simulink model "Function11"  (R2016b)
settings: Solver=VariableStepAuto  StartTime=0.0  StopTime=10.0  RelTol=1e-3
libraries: simulink x2
settings Model: Creator=viett  LastModifiedBy=viett

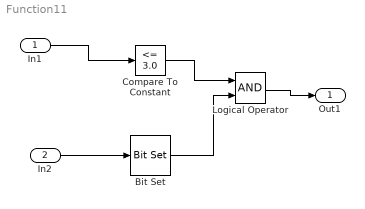
== system Function11 ==
  In1 : Inport
  In2 : Inport  Port=2
  Bit Set : simulink/Logic and Bit Operations/Bit Set  iBit=0
  Compare To Constant : simulink/Logic and Bit Operations/Compare To Constant  relop=<=  const=3.0  OutDataTypeStr=boolean
  Logical Operator : Logic  AllPortsSameDT=off  OutDataTypeStr=boolean
  Out1 : Outport
  wires:
  Compare To Constant/1 -> Logical Operator/1
  Bit Set/1 -> Logical Operator/2
  Logical Operator/1 -> Out1/1
  In1/1 -> Compare To Constant/1
  In2/1 -> Bit Set/1
